simulink model "Solar_cell_char"  (R2020a)
settings: Solver=VariableStepAuto  StartTime=0.0  StopTime=4  RelTol=1e-3
libraries: powerlib x5, simulink x2, re_lib x1
settings Model: Creator=ASUS  LastModifiedBy=ASUS

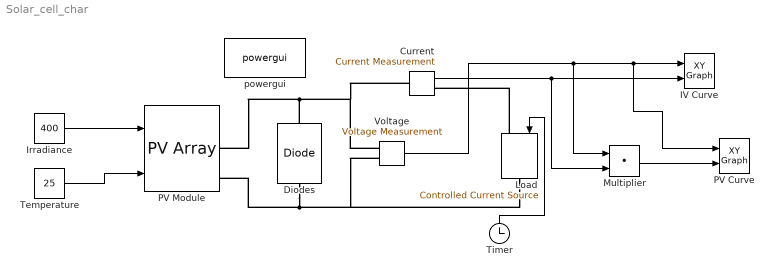
== system Solar_cell_char ==
  Current : powerlib/Measurements/Current Measurement  PhasorSimulation=off  OutputType=Complex  PSBequivalent=0
  Diodes : powerlib/Power Electronics/Diode  Ron=0.001  Lon=0  Vf=0.8  IC=0  UseSnubber=0  Rs=500  Cs=250e-9  Measurements=off
  IV Curve : simulink/Sinks/XY Graph  xmin=0  xmax=25  ymin=0  ymax=9  st=-1
  Irradiance : Constant  Value=400
  Load : powerlib/Electrical Sources/Controlled Current Source  Initialize=on  Source_Type=AC  Amplitude=0  Phase=0  Frequency=0  Measurements=None
  Multiplier : DotProduct  InputSameDT=on  OutDataTypeStr=Inherit: Inherit via internal rule
  PV Curve : simulink/Sinks/XY Graph  xmin=0  xmax=25  ymin=0  ymax=150  st=-1
  PV Module : re_lib/Solar/PV Array  Npar=1  Nser=1  PlotType=array @ 1000 W/m2 & specified temperatures  S_vec="[ 1000  500  100 ]"  Temp_C_vec="[ 45 25  ]"  ModuleName=Luxor Solar Solo Line 140M  PlotWhenSelected=off  Pm=140.0148  Ncell=36  Voc=22.57  Isc=8.97  Vm=17.48  Im=8.01  beta_Voc_pc=-0.32419  alpha_Isc_pc=0.041405  beta_Voc=-0.07317  alpha_Isc=0.003714  IL=9.008  I0=7.8539e-11  nI=0.96087  Rsh=37.2802  Rs=0.311  RobustModel=off  RobustCellTemperature=25  BAL=off  Tc=1e-6  Tfilter=5e-5
  Temperature : Constant  Value=25
  Timer : Clock
  "Voltage " : powerlib/Measurements/Voltage Measurement  PhasorSimulation=off  OutputType=Complex  PSBequivalent=0
  powergui : powerlib/powergui  Priority=1  SimulationMode=Continuous  SampleTime=50e-6  frequency=60  Iterations=50  frequencyindice=0  Pbase=100e6  ErrMax=1e-4  UnitsV=kV  UnitsW=MW  buscounter=0  FunctionMessages=off  echomessages=off  EnableUseOfTLC=off  CurrentSourceSwitches=off  DisableSnubberDevices=off  DisableRonSwitches=off  DisableVfSwitches=off  DisplayEquations=off  AutomaticDiscreteSolvers=off  SolverType=Tustin/Backward Euler (TBE)  Interpol=off  ExternalGateDelay=off  methode=off  Ts=100  x0status=blocks  SPID=on  SwTol=0  HookPort=off  NonlinearTolerance=1e-4  nMaxIteration=100  ContinueOnMaxIteration=off  RestoreLinks=warning  ResistiveCurrentMeasurement=off  Frange=[0:2:500]  Ylog=off  Xlog=on  ShowGrid=off  save=off  variable=ZData  structure=0  ZoomFFT=off  StartTime=0.0  cycles=1  DisplayStyle=1  fundamental=60  FreqAxis=off  MaxFrequency=1000  frequencyindicesteady=1  RmsSteady=1  display=off
  wires:
  Irradiance/1 -> PV Module/1
  Temperature/1 -> PV Module/2
  Current/1 -> Multiplier/2, IV Curve/2
  "Voltage "/1 -> Multiplier/1, PV Curve/1, IV Curve/1
  Multiplier/1 -> PV Curve/2
  Timer/1 -> Load/1
  connections:
  Diodes/RConn1 -- Current/LConn1 -- "Voltage "/LConn1 -- PV Module/RConn1
  Diodes/LConn1 -- Load/RConn1 -- "Voltage "/LConn2 -- PV Module/RConn2
  Load/LConn1 -- Current/RConn1
